simulink model "TST_FlFWLvl_VD"  (R2016b)
settings: Solver=FixedStepDiscrete  StartTime=0.0  StopTime=simTime  FixedStep=sampleTime  RelTol=1e-3
values from neighbouring files (symbols this model uses):
  testCase = 1    [initTST_FlFWLvl_VD_001.m]    (also in initTST_FlFWLvl_VD_002.m = 2)
libraries: simulink x5, UnitTest_Lib x2
settings Model: Creator=zhengjinyan  LastModifiedBy=zhengjinyan
settings DebuggingCC: SignalRangeChecking=error

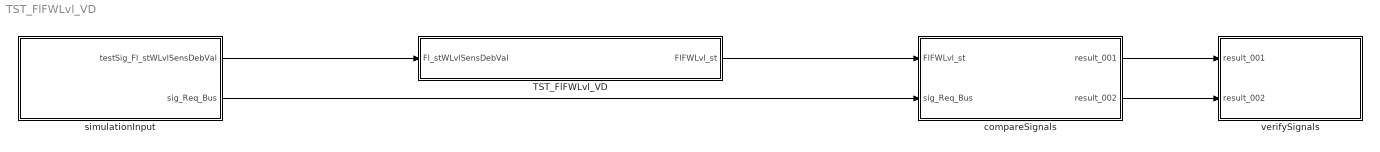
== system TST_FlFWLvl_VD ==
  TST_FlFWLvl_VD : Subsystem
  compareSignals : Subsystem
  simulationInput : Subsystem
  verifySignals : Subsystem
  wires:
  simulationInput/1(testSig_Fl_stWLvlSensDebVal) -> TST_FlFWLvl_VD/1(Fl_stWLvlSensDebVal)
  TST_FlFWLvl_VD/1(FlFWLvl_st) -> compareSignals/1(FlFWLvl_st)
  simulationInput/2(sig_Req_Bus) -> compareSignals/2(sig_Req_Bus)
  compareSignals/1(result_001) -> verifySignals/1(result_001)
  compareSignals/2(result_002) -> verifySignals/2(result_002)

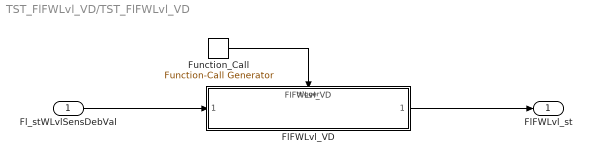
== system TST_FlFWLvl_VD/TST_FlFWLvl_VD ==
  Fl_stWLvlSensDebVal : Inport
  FlFWLvl_VD : ModelReference  ModelNameDialog=FlFWLvl_VD  SimulationMode=Normal  ModelReferenceVersion=1.5  TriggerPortName=function  TriggerPortTriggerType=function-call  TriggerPortStatesWhenEnabling=held
  Function_Call : simulink/Ports & Subsystems/Function-Call Generator  sample_time=sampleTime  numberOfIterations=1
  FlFWLvl_st : Outport
  wires:
  Function_Call/1 -> FlFWLvl_VD/Trigger
  Fl_stWLvlSensDebVal/1 -> FlFWLvl_VD/1
  FlFWLvl_VD/1 -> FlFWLvl_st/1

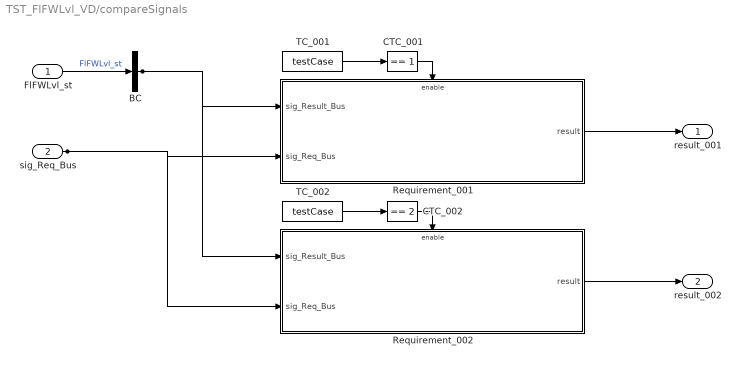
== system TST_FlFWLvl_VD/compareSignals ==
  FlFWLvl_st : Inport
  sig_Req_Bus : Inport  Port=2
  BC : BusCreator  Inputs=1
  CTC_001 : simulink/Logic and Bit Operations/Compare To Constant  relop===  const=1  OutDataTypeStr=boolean
  CTC_002 : simulink/Logic and Bit Operations/Compare To Constant  relop===  const=2  OutDataTypeStr=boolean
  Requirement_001 : Subsystem
  Requirement_002 : Subsystem
  TC_001 : Constant  Value=testCase
  TC_002 : Constant  Value=testCase
  result_001 : Outport
  result_002 : Outport  Port=2
  wires:
  FlFWLvl_st/1 -> BC/1  "FlFWLvl_st"
  TC_001/1 -> CTC_001/1
  CTC_001/1 -> Requirement_001/Enable
  sig_Req_Bus/1 -> Requirement_001/2(sig_Req_Bus), Requirement_002/2(sig_Req_Bus)
  BC/1 -> Requirement_001/1(sig_Result_Bus), Requirement_002/1(sig_Result_Bus)
  Requirement_001/1(result) -> result_001/1
  TC_002/1 -> CTC_002/1
  CTC_002/1 -> Requirement_002/Enable
  Requirement_002/1(result) -> result_002/1

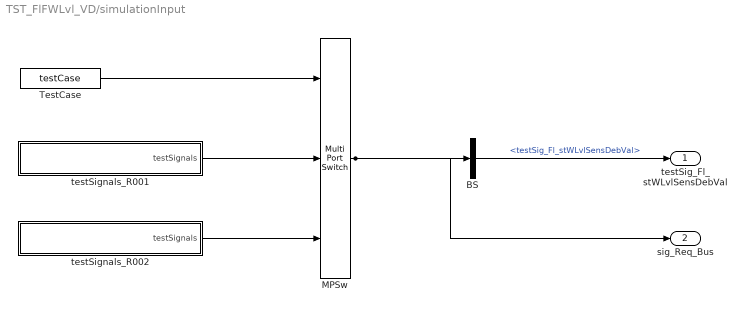
== system TST_FlFWLvl_VD/simulationInput ==
  BS : BusSelector  OutputSignals=testSig_Fl_stWLvlSensDebVal
  MPSw : MultiPortSwitch  Inputs=2  SaturateOnIntegerOverflow=on  InputSameDT=on
  TestCase : Constant  Value=testCase
  testSignals_R001 : Subsystem
  testSignals_R002 : Subsystem
  testSig_Fl_stWLvlSensDebVal : Outport
  sig_Req_Bus : Outport  Port=2
  wires:
  BS/1 -> testSig_Fl_stWLvlSensDebVal/1  "<testSig_Fl_stWLvlSensDebVal>"
  MPSw/1 -> BS/1, sig_Req_Bus/1
  TestCase/1 -> MPSw/1
  testSignals_R001/1(testSignals) -> MPSw/2
  testSignals_R002/1(testSignals) -> MPSw/3

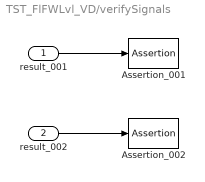
== system TST_FlFWLvl_VD/verifySignals ==
  result_001 : Inport
  result_002 : Inport  Port=2
  Assertion_001 : Assertion  Enabled=off
  Assertion_002 : Assertion  Enabled=off
  wires:
  result_001/1 -> Assertion_001/1
  result_002/1 -> Assertion_002/1

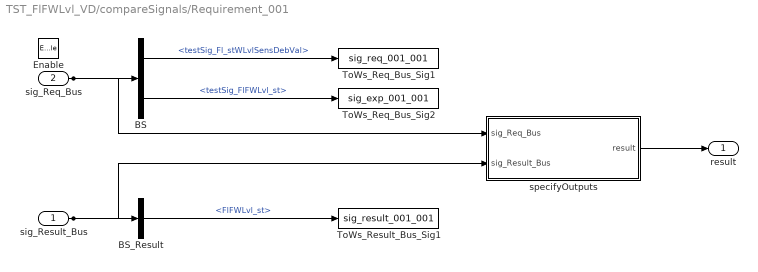
== system TST_FlFWLvl_VD/compareSignals/Requirement_001 ==
  sig_Result_Bus : Inport
  sig_Req_Bus : Inport  Port=2
  Enable : EnablePort
  BS : BusSelector  OutputSignals=testSig_Fl_stWLvlSensDebVal,testSig_FlFWLvl_st
  BS_Result : BusSelector  OutputSignals=FlFWLvl_st
  ToWs_Req_Bus_Sig1 : ToWorkspace  VariableName=sig_req_001_001  SaveFormat=Structure With Time
  ToWs_Req_Bus_Sig2 : ToWorkspace  VariableName=sig_exp_001_001  SaveFormat=Structure With Time
  ToWs_Result_Bus_Sig1 : ToWorkspace  VariableName=sig_result_001_001  SaveFormat=Structure With Time
  specifyOutputs : Subsystem
  result : Outport
  wires:
  sig_Req_Bus/1 -> BS/1, specifyOutputs/1(sig_Req_Bus)
  BS/1 -> ToWs_Req_Bus_Sig1/1  "<testSig_Fl_stWLvlSensDebVal>"
  BS/2 -> ToWs_Req_Bus_Sig2/1  "<testSig_FlFWLvl_st>"
  sig_Result_Bus/1 -> BS_Result/1, specifyOutputs/2(sig_Result_Bus)
  BS_Result/1 -> ToWs_Result_Bus_Sig1/1  "<FlFWLvl_st>"
  specifyOutputs/1(result) -> result/1

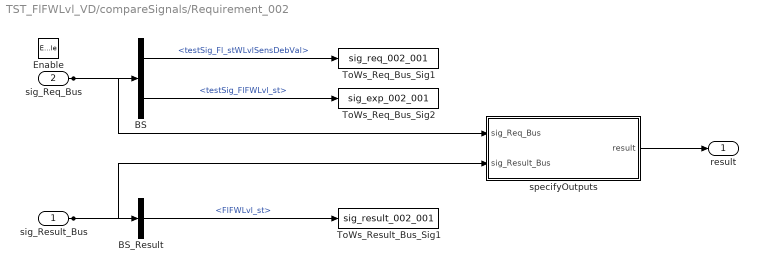
== system TST_FlFWLvl_VD/compareSignals/Requirement_002 ==
  sig_Result_Bus : Inport
  sig_Req_Bus : Inport  Port=2
  Enable : EnablePort
  BS : BusSelector  OutputSignals=testSig_Fl_stWLvlSensDebVal,testSig_FlFWLvl_st
  BS_Result : BusSelector  OutputSignals=FlFWLvl_st
  ToWs_Req_Bus_Sig1 : ToWorkspace  VariableName=sig_req_002_001  SaveFormat=Structure With Time
  ToWs_Req_Bus_Sig2 : ToWorkspace  VariableName=sig_exp_002_001  SaveFormat=Structure With Time
  ToWs_Result_Bus_Sig1 : ToWorkspace  VariableName=sig_result_002_001  SaveFormat=Structure With Time
  specifyOutputs : Subsystem
  result : Outport
  wires:
  sig_Req_Bus/1 -> BS/1, specifyOutputs/1(sig_Req_Bus)
  BS/1 -> ToWs_Req_Bus_Sig1/1  "<testSig_Fl_stWLvlSensDebVal>"
  BS/2 -> ToWs_Req_Bus_Sig2/1  "<testSig_FlFWLvl_st>"
  sig_Result_Bus/1 -> BS_Result/1, specifyOutputs/2(sig_Result_Bus)
  BS_Result/1 -> ToWs_Result_Bus_Sig1/1  "<FlFWLvl_st>"
  specifyOutputs/1(result) -> result/1

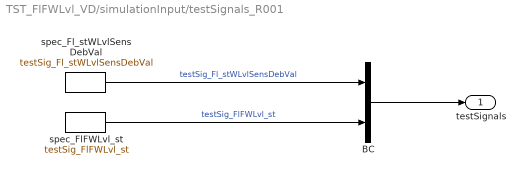
== system TST_FlFWLvl_VD/simulationInput/testSignals_R001 ==
  BC : BusCreator  Inputs=2
  spec_FlFWLvl_st : FromWorkspace  VariableName=testSig_FlFWLvl_st  Interpolate=off  OutputAfterFinalValue=Holding final value
  spec_Fl_stWLvlSensDebVal : FromWorkspace  VariableName=testSig_Fl_stWLvlSensDebVal  Interpolate=off  OutputAfterFinalValue=Holding final value
  testSignals : Outport
  wires:
  BC/1 -> testSignals/1
  spec_Fl_stWLvlSensDebVal/1 -> BC/1  "testSig_Fl_stWLvlSensDebVal"
  spec_FlFWLvl_st/1 -> BC/2  "testSig_FlFWLvl_st"

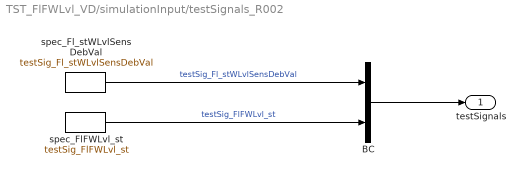
== system TST_FlFWLvl_VD/simulationInput/testSignals_R002 ==
  BC : BusCreator  Inputs=2
  spec_FlFWLvl_st : FromWorkspace  VariableName=testSig_FlFWLvl_st  Interpolate=off  OutputAfterFinalValue=Holding final value
  spec_Fl_stWLvlSensDebVal : FromWorkspace  VariableName=testSig_Fl_stWLvlSensDebVal  Interpolate=off  OutputAfterFinalValue=Holding final value
  testSignals : Outport
  wires:
  BC/1 -> testSignals/1
  spec_Fl_stWLvlSensDebVal/1 -> BC/1  "testSig_Fl_stWLvlSensDebVal"
  spec_FlFWLvl_st/1 -> BC/2  "testSig_FlFWLvl_st"

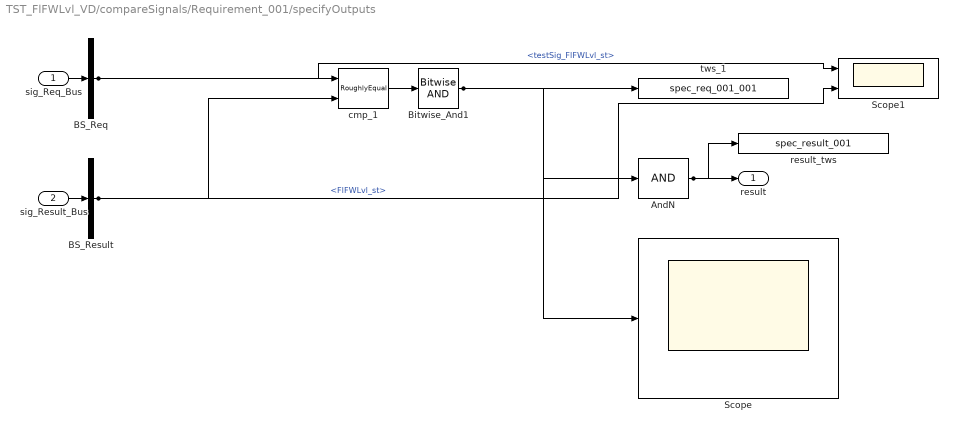
== system TST_FlFWLvl_VD/compareSignals/Requirement_001/specifyOutputs ==
  sig_Req_Bus : Inport
  sig_Result_Bus : Inport  Port=2
  AndN : Logic  Inputs=1
  BS_Req : BusSelector  OutputSignals=testSig_FlFWLvl_st
  BS_Result : BusSelector  OutputSignals=FlFWLvl_st
  Bitwise_And1 : simulink/Logic and Bit Operations/Bitwise Operator  logicop=AND  UseBitMask=off  BitMask=bin2dec('11011001')  BitMaskRealWorld=Stored Integer
  Scope : Scope
  Scope1 : Scope  NumInputPorts=2
  cmp_1 : UnitTest_Lib/RoughlyEqual  slope=0.1
  result_tws : ToWorkspace  VariableName=spec_result_001
  tws_1 : ToWorkspace  VariableName=spec_req_001_001
  result : Outport
  wires:
  sig_Req_Bus/1 -> BS_Req/1
  sig_Result_Bus/1 -> BS_Result/1
  AndN/1 -> result/1, result_tws/1
  BS_Req/1 -> cmp_1/1, Scope1/1  "<testSig_FlFWLvl_st>"
  BS_Result/1 -> cmp_1/2, Scope1/2  "<FlFWLvl_st>"
  cmp_1/1 -> Bitwise_And1/1
  Bitwise_And1/1 -> tws_1/1, AndN/1, Scope/1

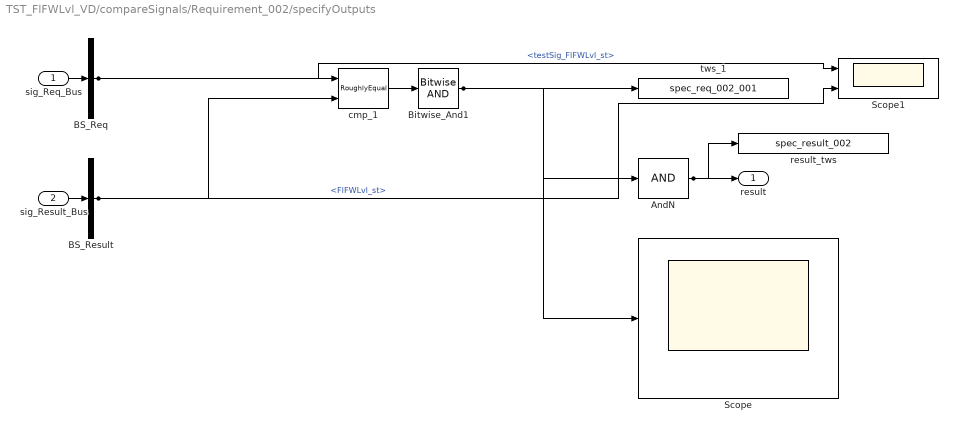
== system TST_FlFWLvl_VD/compareSignals/Requirement_002/specifyOutputs ==
  sig_Req_Bus : Inport
  sig_Result_Bus : Inport  Port=2
  AndN : Logic  Inputs=1
  BS_Req : BusSelector  OutputSignals=testSig_FlFWLvl_st
  BS_Result : BusSelector  OutputSignals=FlFWLvl_st
  Bitwise_And1 : simulink/Logic and Bit Operations/Bitwise Operator  logicop=AND  UseBitMask=off  BitMask=bin2dec('11011001')  BitMaskRealWorld=Stored Integer
  Scope : Scope
  Scope1 : Scope  NumInputPorts=2
  cmp_1 : UnitTest_Lib/RoughlyEqual  slope=0.1
  result_tws : ToWorkspace  VariableName=spec_result_002
  tws_1 : ToWorkspace  VariableName=spec_req_002_001
  result : Outport
  wires:
  sig_Req_Bus/1 -> BS_Req/1
  sig_Result_Bus/1 -> BS_Result/1
  AndN/1 -> result/1, result_tws/1
  BS_Req/1 -> cmp_1/1, Scope1/1  "<testSig_FlFWLvl_st>"
  BS_Result/1 -> cmp_1/2, Scope1/2  "<FlFWLvl_st>"
  cmp_1/1 -> Bitwise_And1/1
  Bitwise_And1/1 -> tws_1/1, AndN/1, Scope/1
